simulink model "AutoRS_Simulation"  (R2022b)
settings: Solver=FixedStepAuto  StartTime=0.0  StopTime=50  FixedStep=1/10e4  RelTol=1e-3
values from neighbouring files (symbols this model uses):
  beta_array = [0 0.0872664625997 0.174532925199 0.261799387799 0.349065850399 0.436332312999 0.523598775598 0.698131700798 0.872664625997 1.0471975512 1.2217304764 1.3962634016 ... (13 elements, 1x13)]    [CQ_CT_maps.mat]
  CQ_entries = [0.00463492513935 0.0049015417371 0.00516815833485 0.00555696036228 0.0059457623897 0.00611397686765 0.00628219134561 0.012914252991 0.0255245334589 0.0349006692545 0.0430149587943 0.0524658396931 ... (507 elements, 39x13)]    [CQ_CT_maps.mat]
  CT_entries = [0.0686211548678 0.0728422059393 0.0770632570108 0.0836290674204 0.09019487783 0.0932108047116 0.0962267315932 0.135717354129 0.192838891055 0.239446349533 0.288110808378 0.351656989082 ... (507 elements, 39x13)]    [CQ_CT_maps.mat]
  lambda_array = [0 0.25 0.5 0.75 1 1.25 1.5 2 2.5 3 3.5 4 ... (39 elements, 39x1)]    [CQ_CT_maps.mat]
undefined symbols (not defined in the file or in its folder): c
settings Model: Creator=Aaron  LastModifiedBy=Sebastian
settings DebuggingCC: UnconnectedInputMsg=warning  UnconnectedOutputMsg=warning  UnconnectedLineMsg=warning
settings ModelReferenceCC: EnableRefExpFcnMdlSchedulingChecks=on
settings RTWCC: DLArmComputeVersion=19.05

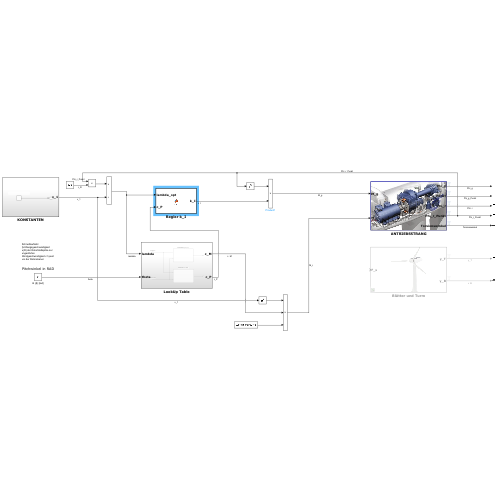
[thumbnail: Simulink's stored preview of the top-level diagram]
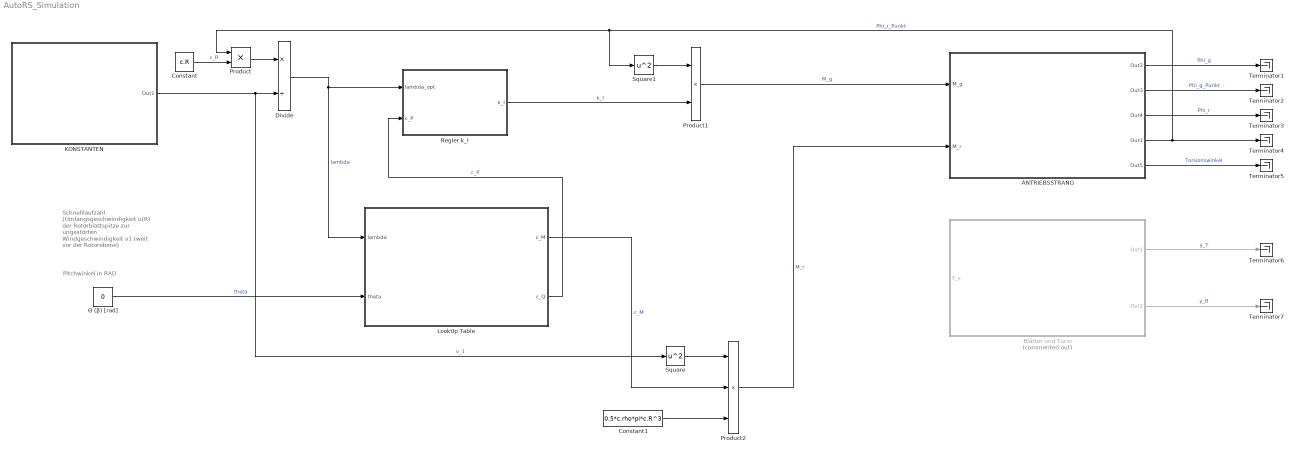
== system AutoRS_Simulation ==
  note: Schnelllaufzahl
      | (Umfangsgeschwindigkeit u(R) der Rotorblattspitze zur ungestörten Windgeschwindigkeit v1 (weit vor der Rotorebene)
  note: Pitchwinkel in RAD
  ANTRIEBSSTRANG : Subsystem
      mask Display: image('C:\Users\Sebastian\Desktop\AutoRS\3. Bilder\Simulink\Antriebsstrang.jpg'); % Use "Edit Image" on toolstrip to change.
  Blätter und Turm : Subsystem  Commented=on
      mask Display: image('C:\Users\Sebastian\Desktop\AutoRS\3. Bilder\Simulink\Blatt_und_Turm'); % Use "Edit Image" on toolstrip to change.
  Constant : Constant  Value=c.R
  Constant1 : Constant  Value=0.5*c.rho*pi*c.R^3
  Divide : Product  Inputs=*/
  KONSTANTEN : Subsystem
  LookUp Table : Subsystem
  Product : Product
  Product1 : Product
  Product2 : Product  Inputs=3
  Regler k_I : MATLAB Function  TreatAsAtomicUnit=on
  Square : Math  Operator=square
  Square1 : Math  Operator=square
  Terminator{1..7} (7 alike) : Terminator
  Θ (β) [rad] : Constant  Value=0
  wires:
  Divide/1 -> LookUp Table/1(lambda), Regler k_I/1(lambda_opt)  "lambda"
  Θ (β) [rad]/1 -> LookUp Table/2(theta)  "theta"
  ANTRIEBSSTRANG/1(Out2) -> Terminator1/1  "Phi_g"
  ANTRIEBSSTRANG/2(Out3) -> Terminator2/1  "Phi_g_Punkt"
  ANTRIEBSSTRANG/3(Out4) -> Terminator3/1  "Phi_r"
  ANTRIEBSSTRANG/4(Out1) -> Square1/1, Product/1, Terminator4/1  "Phi_r_Punkt"
  ANTRIEBSSTRANG/5(Out5) -> Terminator5/1  "Torsionswinkel"
  Blätter und Turm/1(Out1) -> Terminator6/1  "y_T"
  Blätter und Turm/2(Out2) -> Terminator7/1  "y_B"
  Product/1 -> Divide/1
  Constant/1 -> Product/2  "c_R"
  KONSTANTEN/1(Out1) -> Square/1, Divide/2  "v_1"
  LookUp Table/1(c_M) -> Product2/2  "c_M"
  Product1/1 -> ANTRIEBSSTRANG/1(M_g)  "M_g"
  Constant1/1 -> Product2/3
  Square/1 -> Product2/1
  Product2/1 -> ANTRIEBSSTRANG/2(M_r)  "M_r"
  Square1/1 -> Product1/1
  LookUp Table/2(c_Q) -> Regler k_I/2(c_P)  "c_P"
  Regler k_I/1(k_I) -> Product1/2  "k_I"

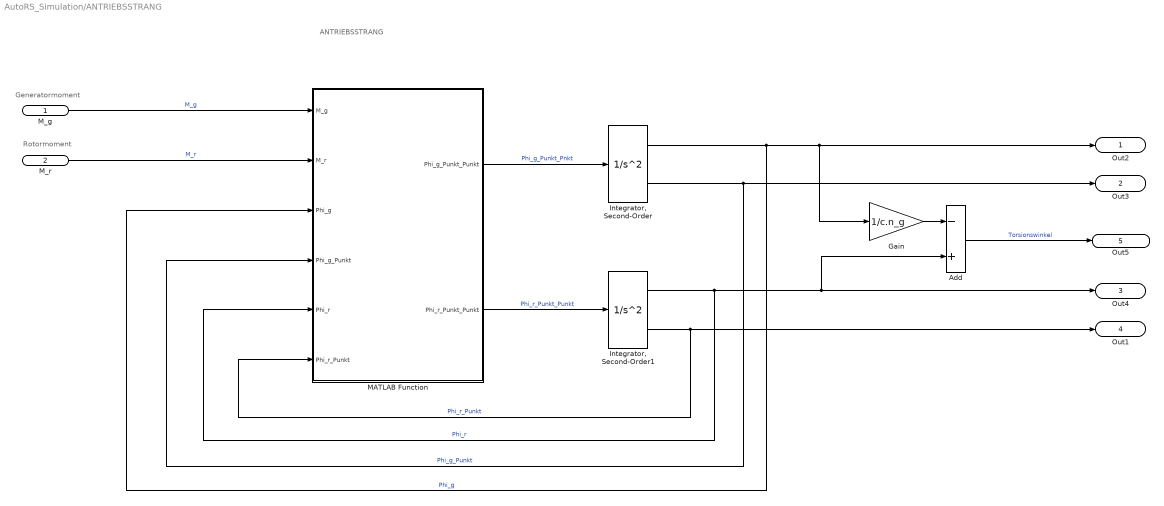
== system AutoRS_Simulation/ANTRIEBSSTRANG ==
  note: ANTRIEBSSTRANG
  note: Rotormoment
  note: Generatormoment
  M_g : Inport
  M_r : Inport  Port=2
  Add : Sum  Inputs=-+
  Gain : Gain  Gain=1/c.n_g
  "Integrator, Second-Order" : SecondOrderIntegrator
  "Integrator, Second-Order1" : SecondOrderIntegrator
  MATLAB Function : MATLAB Function  TreatAsAtomicUnit=on
  Out2 : Outport
  Out3 : Outport  Port=2
  Out4 : Outport  Port=3
  Out1 : Outport  Port=4
  Out5 : Outport  Port=5
  wires:
  "Integrator, Second-Order1"/2 -> Out1/1, MATLAB Function/6(Phi_r_Punkt)  "Phi_r_Punkt"
  "Integrator, Second-Order1"/1 -> Out4/1, Add/2, MATLAB Function/5(Phi_r)  "Phi_r"
  MATLAB Function/1(Phi_g_Punkt_Punkt) -> "Integrator, Second-Order"/1  "Phi_g_Punkt_Pnkt"
  "Integrator, Second-Order"/1 -> Out2/1, Gain/1, MATLAB Function/3(Phi_g)  "Phi_g"
  "Integrator, Second-Order"/2 -> Out3/1, MATLAB Function/4(Phi_g_Punkt)  "Phi_g_Punkt"
  Add/1 -> Out5/1  "Torsionswinkel"
  M_g/1 -> MATLAB Function/1(M_g)  "M_g"
  M_r/1 -> MATLAB Function/2(M_r)  "M_r"
  MATLAB Function/2(Phi_r_Punkt_Punkt) -> "Integrator, Second-Order1"/1  "Phi_r_Punkt_Punkt"
  Gain/1 -> Add/1

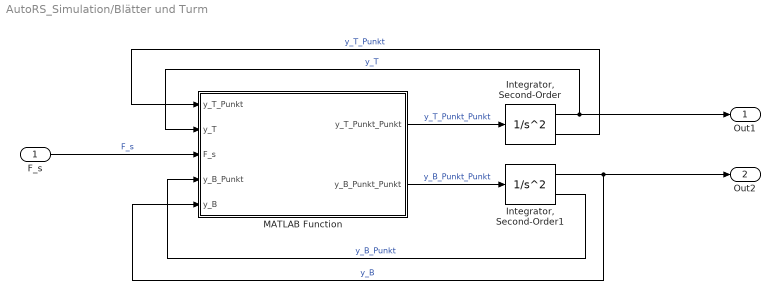
== system AutoRS_Simulation/Blätter und Turm ==
  F_s : Inport
  "Integrator, Second-Order" : SecondOrderIntegrator  ICX=0
  "Integrator, Second-Order1" : SecondOrderIntegrator  ICX=0
  MATLAB Function : MATLAB Function  TreatAsAtomicUnit=on
  Out1 : Outport
  Out2 : Outport  Port=2
  wires:
  MATLAB Function/2(y_B_Punkt_Punkt) -> "Integrator, Second-Order1"/1  "y_B_Punkt_Punkt"
  MATLAB Function/1(y_T_Punkt_Punkt) -> "Integrator, Second-Order"/1  "y_T_Punkt_Punkt"
  "Integrator, Second-Order"/1 -> Out1/1, MATLAB Function/2(y_T)  "y_T"
  F_s/1 -> MATLAB Function/3(F_s)  "F_s"
  "Integrator, Second-Order"/2 -> MATLAB Function/1(y_T_Punkt)  "y_T_Punkt"
  "Integrator, Second-Order1"/2 -> MATLAB Function/4(y_B_Punkt)  "y_B_Punkt"
  "Integrator, Second-Order1"/1 -> Out2/1, MATLAB Function/5(y_B)  "y_B"

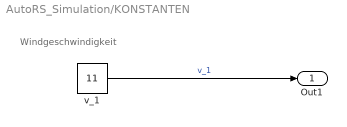
== system AutoRS_Simulation/KONSTANTEN ==
  note: Windgeschwindigkeit
  v_1 : Constant  Value=11
  Out1 : Outport
  wires:
  v_1/1 -> Out1/1  "v_1"

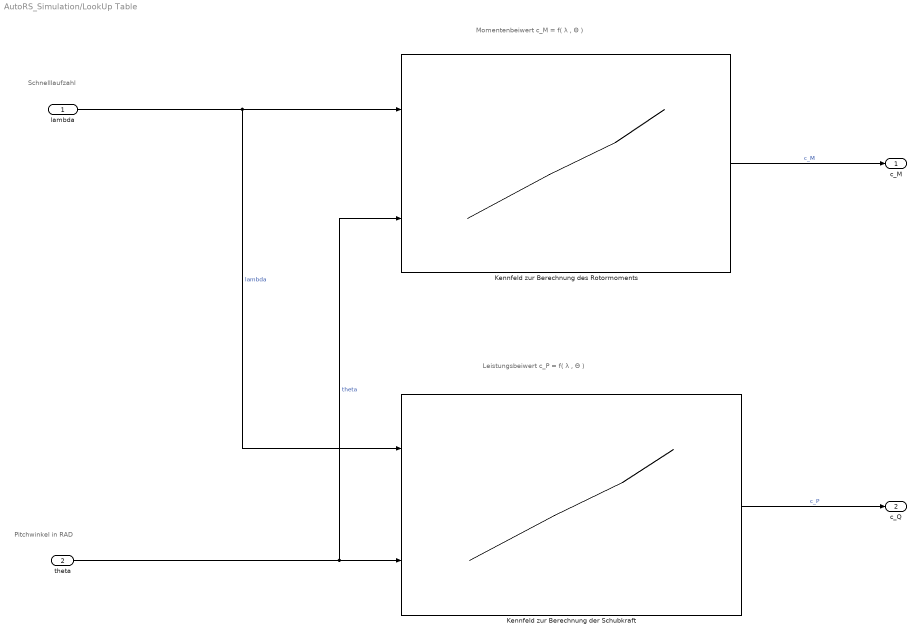
== system AutoRS_Simulation/LookUp Table ==
  note: Schnelllaufzahl
  note: Pitchwinkel in RAD
  note: Momentenbeiwert c_M = f( λ , Θ )
  note: Leistungsbeiwert c_P = f( λ , Θ )
  lambda : Inport
  theta : Inport  Port=2
  Kennfeld zur Berechnung der Schubkraft : Lookup_n-D  BreakpointsForDimension1=lambda_array  BreakpointsForDimension2=beta_array  Table=CT_entries  InternalRulePriority=Speed  RndMeth=Simplest
      settings: InputPortMap=u0,u1
  Kennfeld zur Berechnung des Rotormoments : Lookup_n-D  BreakpointsForDimension1=lambda_array  BreakpointsForDimension2=beta_array  Table=CQ_entries  InternalRulePriority=Speed  RndMeth=Simplest
      settings: InputPortMap=u0,u1
  c_M : Outport
  c_Q : Outport  Port=2
  wires:
  Kennfeld zur Berechnung der Schubkraft/1 -> c_Q/1  "c_P"
  Kennfeld zur Berechnung des Rotormoments/1 -> c_M/1  "c_M"
  lambda/1 -> Kennfeld zur Berechnung des Rotormoments/1, Kennfeld zur Berechnung der Schubkraft/1  "lambda"
  theta/1 -> Kennfeld zur Berechnung des Rotormoments/2, Kennfeld zur Berechnung der Schubkraft/2  "theta"

== matlab function AutoRS_Simulation/Blätter und Turm/MATLAB Function ==
  data: y_T_Punkt input; y_T input; F_s input; y_T_Punkt_Punkt output; y_B_Punkt input; y_B input; y_B_Punkt_Punkt output
function [y_T_Punkt_Punkt, y_B_Punkt_Punkt] = fcn(y_T_Punkt, y_T, F_s, y_B_Punkt, y_B)

    % KONSTANTEN AUFRUFEN
    c = Konstanten();
    
    % BERECHNUNG
    y_T_Punkt_Punkt = (-c.k_T*y_T-c.d_T*y_T_Punkt+3*c.k_B*(y_B-y_T)+3*c.d_B*(y_B_Punkt-y_T_Punkt))/c.m_T;
    
    y_B_Punkt_Punkt = (-3*c.k_B*(y_B-y_T)-3*c.d_B*(y_B_Punkt-y_T_Punkt)+F_s)/(3*c.m_B);
end

== matlab function AutoRS_Simulation/ANTRIEBSSTRANG/MATLAB Function ==
  data: M_g input; M_r input; Phi_g_Punkt_Punkt output; Phi_r_Punkt_Punkt output; Phi_g input; Phi_g_Punkt input; Phi_r input; Phi_r_Punkt input
function [Phi_g_Punkt_Punkt, Phi_r_Punkt_Punkt]= fcn(M_g, M_r, Phi_g, Phi_g_Punkt, Phi_r, Phi_r_Punkt)
    
    % KONSTANTEN AUFRUFEN
    c = Konstanten();

    % BERECHNUNGEN
    Phi_g_Punkt_Punkt = (-c.k_s*(Phi_g-c.n_g*Phi_r)-c.d_s*(Phi_g_Punkt-c.n_g*Phi_r_Punkt)-M_g)/c.J_g;

    Phi_r_Punkt_Punkt = (M_r-c.n_g*(c.k_s*(c.n_g*Phi_r-Phi_g))-c.n_g*(c.d_s*(c.n_g*Phi_r_Punkt-Phi_g_Punkt)))/c.J_r;
end

== matlab function AutoRS_Simulation/Regler k_I ==
  data: lambda_opt input; k_I output; c_P input
function k_I = fcn(lambda_opt, c_P)

    % KONSTANTEN AUFRUFEN
    c = Konstanten();

    % BERECHNUNG
    k_I = 0.5*c.rho*pi*c.R^5*1/lambda_opt^3*1/c.n_g^3*c_P;
end
